simulink model "TorqueVect"  (R2022a)
settings: Solver=VariableStepAuto  StartTime=0.0  StopTime=32  RelTol=1e-3
PreLoadFcn:
  | run('Parameters\FSE_Parameters.m')
undefined symbols (not defined in the file): BRegenEnabledButton, canChannel, CyalphaLookUp, efficiency, Fz_curve, Fz_scaling_long, gearR, izz, jw, Kd, kd, Ki, ki, Kp, kp, l_f, l_r, lambda, m, Mz_max, N, N_lat, N_long, P_max, pid_kd_lat, pid_kd_long, pid_ki_lat, pid_ki_long, pid_kp_lat, pid_kp_long, R_max, rw, steerR, T_i_max, TC_Decr_Gas, TC_Derivative, TC_Incr_Gas, TC_On, TC_Relay_Off, TC_Relay_On, tireCornerStiffness, Ts, TV_On, TV_Override, velocity_lookup, velocity_lookup_lat, y_ref, yrr_scaling
libraries: simulink x218, slpidlib x135, CarMaker4SL x101, TractionControlLibrary x13, canmsglib x9, canlib x8, TorqueVectoringLibrary x6, simulink_extras x4, PedalConversionLibrary x3, PowerControlLibrary x1
(part 21 of 26)

== system TorqueVect/CarMaker/IPG Vehicle/PowerTrain/PTControl Example/PTControl_ALL_CTRL_VC_REGEN/Subsystem/TC/TractionControlFR/PID Controller ==
  rSlipError : Inport
  BEnable_TC : Inport  Port=2
  Kp_TC : Inport  Port=3
  Kd_TC : Inport  Port=4
  Ki_TC : Inport  Port=5
  MMotorMax : Inport  Port=6
  Constant : Constant  Value=0
  Constant1 : Constant  Value=0
  PID Controller : slpidlib/PID Controller  Controller=PID  Form=Ideal  TimeDomain=Discrete-time  UseExternalTs=off  SampleTime=0.005  IntegratorMethod=Forward Euler  FilterMethod=Forward Euler  ControllerParametersSource=external  P=Kp  I=Ki  UseKiTs=on  D=Kd  N=100  UseFilter=off  TunerSelectOption=Transfer Function Based (PID Tuner App)  InitialConditionSource=internal  InitialConditionForIntegrator=0  InitialConditionForFilter=0  DifferentiatorICPrevScaledInput=0  ExternalReset=either  TrackingMode=off  Kt=1  LimitOutput=on  SatLimitsSource=external  UpperSaturationLimit=21  LowerSaturationLimit=0  LinearizeAsGain=on  AntiWindupMode=none  Kb=1  POutMin=[]  POutMax=[]  IOutMin=[]  IOutMax=[]  DOutMin=[]  DOutMax=[]  NOutMin=[]  NOutMax=[]  SumOutMin=[]  SumOutMax=[]  SaturationOutMin=[]  SaturationOutMax=[]  PParamMin=[]  PParamMax=[]  IParamMin=[]  IParamMax=[]  DParamMin=[]  DParamMax=[]  NParamMin=[]  NParamMax=[]  KbParamMin=[]  KbParamMax=[]  KtParamMin=[]  KtParamMax=[]  KbOutMin=[]  KbOutMax=[]  KtOutMin=[]  KtOutMax=[]  IntegratorOutMin=[]  IntegratorOutMax=[]  FilterOutMin=[]  FilterOutMax=[]  SumI1OutMin=[]  SumI1OutMax=[]  SumI2OutMin=[]  SumI2OutMax=[]  SumI3OutMin=[]  SumI3OutMax=[]  SumI4OutMin=[]  SumI4OutMax=[]  SumDOutMin=[]  SumDOutMax=[]  DifferentiatorOutMin=[]  DifferentiatorOutMax=[]  FilterDiffOutCoefMin=[]  FilterDiffOutCoefMax=[]  ReciprocalOutMin=[]  ReciprocalOutMax=[]  SumDenOutMin=[]  SumDenOutMax=[]  SumNumOutMin=[]  SumNumOutMax=[]  DivideOutMin=[]  DivideOutMax=[]  UdiffTsProdOutMin=[]  UdiffTsProdOutMax=[]  NTsProdOutMin=[]  NTsProdOutMax=[]  UintegralTsProdOutMin=[]  UintegralTsProdOutMax=[]  UngainTsProdOutMin=[]  UngainTsProdOutMax=[]  ClampingZeroOutDataTypeStr=Inherit: Inherit via back propagation  ClampingZeroOutMin=[]  ClampingZeroOutMax=[]  FilterDenConstantOutDataTypeStr=Inherit: Inherit via back propagation  FilterDenConstantOutMin=[]  FilterDenConstantOutMax=[]  PCopyOutDataTypeStr=Inherit: Inherit via back propagation  PCopyOutMin=[]  PCopyOutMax=[]  NCopyOutDataTypeStr=Inherit: Inherit via back propagation  NCopyOutMin=[]  NCopyOutMax=[]  IntegratorContinuousStateAttributes=''  IntegratorStateMustResolveToSignalObject=off  IntegratorRTWStateStorageClass=Auto  FilterContinuousStateAttributes=''  FilterStateMustResolveToSignalObject=off  FilterRTWStateStorageClass=Auto  ParallelPVariant=Passthrough  IdealPVariant=ExternalParameters  IVariant=ExternalParameters  DVariant=ExternalParameters  IntegratorVariant=Discrete  SatVariant=External  AWVariant=Passthrough  PCopyVariant=Disabled  TRVariant=Disabled  FdbkBlocksVariant=Forward  IdealPFdbkVariant=Disabled  SatFdbkVariant=Disabled  DerivativeFilterVariant=Differentiator  NVariant=Passthrough  NCopyVariant=Disabled_SignalSpec  FilterICVariant=InternalICsDifferentiator  IntegratorICVariant=InternalICs  ExternalResetVariant=ExternalReset  TRSumVariant=Passthrough  SumFdbkVariant=Disabled  SumVariant=Sum_PID  TsampFilterVariant=InternalTs  TsampNgainVariant=Passthrough  TsampIntegralVariant=Passthrough  ExternalSaturationOutDataTypeStr=Inherit: Same as second input  aMode=0
  Switch : Switch  Criteria=u2 > Threshold  SaturateOnIntegerOverflow=off  InputSameDT=off
  MMotorReduction : Outport  VectorParamsAs1DForOutWhenUnconnected=off
  wires:
  Constant/1 -> Switch/3
  BEnable_TC/1 -> PID Controller/5, Switch/2
  Kp_TC/1 -> PID Controller/2
  rSlipError/1 -> PID Controller/1
  Kd_TC/1 -> PID Controller/4
  Switch/1 -> MMotorReduction/1
  Ki_TC/1 -> PID Controller/3
  Constant1/1 -> PID Controller/7
  MMotorMax/1 -> PID Controller/6
  PID Controller/1 -> Switch/1

== system TorqueVect/CarMaker/IPG Vehicle/PowerTrain/PTControl Example/PTControl_ALL_CTRL_VC_REGEN/Subsystem/TC/TractionControlRL/If Action Subsystem ==
  MMotorRequest : Inport
  Action Port : ActionPort
  Out1 : Outport
  wires:
  MMotorRequest/1 -> Out1/1

== system TorqueVect/CarMaker/IPG Vehicle/PowerTrain/PTControl Example/PTControl_ALL_CTRL_VC_REGEN/Subsystem/TC/TractionControlRL/If Action Subsystem1 ==
  Action Port : ActionPort
  Constant : Constant  Value=0
  Out1 : Outport
  wires:
  Constant/1 -> Out1/1

== system TorqueVect/CarMaker/IPG Vehicle/PowerTrain/PTControl Example/PTControl_ALL_CTRL_VC_REGEN/Subsystem/TC/TractionControlRL/If Action Subsystem2 ==
  MMotorRequest : Inport
  In2 : Inport  Port=2
  Action Port : ActionPort
  Add : Sum  Inputs=+-
  Out1 : Outport
  wires:
  In2/1 -> Add/2
  MMotorRequest/1 -> Add/1
  Add/1 -> Out1/1

== system TorqueVect/CarMaker/IPG Vehicle/PowerTrain/PTControl Example/PTControl_ALL_CTRL_VC_REGEN/Subsystem/TC/TractionControlRL/PID Controller ==
  rSlipError : Inport
  BEnable_TC : Inport  Port=2
  Kp_TC : Inport  Port=3
  Kd_TC : Inport  Port=4
  Ki_TC : Inport  Port=5
  MMotorMax : Inport  Port=6
  Constant : Constant  Value=0
  Constant1 : Constant  Value=0
  PID Controller : slpidlib/PID Controller  Controller=PID  Form=Ideal  TimeDomain=Discrete-time  UseExternalTs=off  SampleTime=0.005  IntegratorMethod=Forward Euler  FilterMethod=Forward Euler  ControllerParametersSource=external  P=Kp  I=Ki  UseKiTs=on  D=Kd  N=100  UseFilter=off  TunerSelectOption=Transfer Function Based (PID Tuner App)  InitialConditionSource=internal  InitialConditionForIntegrator=0  InitialConditionForFilter=0  DifferentiatorICPrevScaledInput=0  ExternalReset=either  TrackingMode=off  Kt=1  LimitOutput=on  SatLimitsSource=external  UpperSaturationLimit=21  LowerSaturationLimit=0  LinearizeAsGain=on  AntiWindupMode=none  Kb=1  POutMin=[]  POutMax=[]  IOutMin=[]  IOutMax=[]  DOutMin=[]  DOutMax=[]  NOutMin=[]  NOutMax=[]  SumOutMin=[]  SumOutMax=[]  SaturationOutMin=[]  SaturationOutMax=[]  PParamMin=[]  PParamMax=[]  IParamMin=[]  IParamMax=[]  DParamMin=[]  DParamMax=[]  NParamMin=[]  NParamMax=[]  KbParamMin=[]  KbParamMax=[]  KtParamMin=[]  KtParamMax=[]  KbOutMin=[]  KbOutMax=[]  KtOutMin=[]  KtOutMax=[]  IntegratorOutMin=[]  IntegratorOutMax=[]  FilterOutMin=[]  FilterOutMax=[]  SumI1OutMin=[]  SumI1OutMax=[]  SumI2OutMin=[]  SumI2OutMax=[]  SumI3OutMin=[]  SumI3OutMax=[]  SumI4OutMin=[]  SumI4OutMax=[]  SumDOutMin=[]  SumDOutMax=[]  DifferentiatorOutMin=[]  DifferentiatorOutMax=[]  FilterDiffOutCoefMin=[]  FilterDiffOutCoefMax=[]  ReciprocalOutMin=[]  ReciprocalOutMax=[]  SumDenOutMin=[]  SumDenOutMax=[]  SumNumOutMin=[]  SumNumOutMax=[]  DivideOutMin=[]  DivideOutMax=[]  UdiffTsProdOutMin=[]  UdiffTsProdOutMax=[]  NTsProdOutMin=[]  NTsProdOutMax=[]  UintegralTsProdOutMin=[]  UintegralTsProdOutMax=[]  UngainTsProdOutMin=[]  UngainTsProdOutMax=[]  ClampingZeroOutDataTypeStr=Inherit: Inherit via back propagation  ClampingZeroOutMin=[]  ClampingZeroOutMax=[]  FilterDenConstantOutDataTypeStr=Inherit: Inherit via back propagation  FilterDenConstantOutMin=[]  FilterDenConstantOutMax=[]  PCopyOutDataTypeStr=Inherit: Inherit via back propagation  PCopyOutMin=[]  PCopyOutMax=[]  NCopyOutDataTypeStr=Inherit: Inherit via back propagation  NCopyOutMin=[]  NCopyOutMax=[]  IntegratorContinuousStateAttributes=''  IntegratorStateMustResolveToSignalObject=off  IntegratorRTWStateStorageClass=Auto  FilterContinuousStateAttributes=''  FilterStateMustResolveToSignalObject=off  FilterRTWStateStorageClass=Auto  ParallelPVariant=Passthrough  IdealPVariant=ExternalParameters  IVariant=ExternalParameters  DVariant=ExternalParameters  IntegratorVariant=Discrete  SatVariant=External  AWVariant=Passthrough  PCopyVariant=Disabled  TRVariant=Disabled  FdbkBlocksVariant=Forward  IdealPFdbkVariant=Disabled  SatFdbkVariant=Disabled  DerivativeFilterVariant=Differentiator  NVariant=Passthrough  NCopyVariant=Disabled_SignalSpec  FilterICVariant=InternalICsDifferentiator  IntegratorICVariant=InternalICs  ExternalResetVariant=ExternalReset  TRSumVariant=Passthrough  SumFdbkVariant=Disabled  SumVariant=Sum_PID  TsampFilterVariant=InternalTs  TsampNgainVariant=Passthrough  TsampIntegralVariant=Passthrough  ExternalSaturationOutDataTypeStr=Inherit: Same as second input  aMode=0
  Switch : Switch  Criteria=u2 > Threshold  SaturateOnIntegerOverflow=off  InputSameDT=off
  MMotorReduction : Outport  VectorParamsAs1DForOutWhenUnconnected=off
  wires:
  Constant/1 -> Switch/3
  BEnable_TC/1 -> PID Controller/5, Switch/2
  Kp_TC/1 -> PID Controller/2
  rSlipError/1 -> PID Controller/1
  Kd_TC/1 -> PID Controller/4
  Switch/1 -> MMotorReduction/1
  Ki_TC/1 -> PID Controller/3
  Constant1/1 -> PID Controller/7
  MMotorMax/1 -> PID Controller/6
  PID Controller/1 -> Switch/1

== system TorqueVect/CarMaker/IPG Vehicle/PowerTrain/PTControl Example/PTControl_ALL_CTRL_VC_REGEN/Subsystem/TC/TractionControlRR/If Action Subsystem ==
  MMotorRequest : Inport
  Action Port : ActionPort
  Out1 : Outport
  wires:
  MMotorRequest/1 -> Out1/1

== system TorqueVect/CarMaker/IPG Vehicle/PowerTrain/PTControl Example/PTControl_ALL_CTRL_VC_REGEN/Subsystem/TC/TractionControlRR/If Action Subsystem1 ==
  Action Port : ActionPort
  Constant : Constant  Value=0
  Out1 : Outport
  wires:
  Constant/1 -> Out1/1

== system TorqueVect/CarMaker/IPG Vehicle/PowerTrain/PTControl Example/PTControl_ALL_CTRL_VC_REGEN/Subsystem/TC/TractionControlRR/If Action Subsystem2 ==
  MMotorRequest : Inport
  In2 : Inport  Port=2
  Action Port : ActionPort
  Add : Sum  Inputs=+-
  Out1 : Outport
  wires:
  In2/1 -> Add/2
  MMotorRequest/1 -> Add/1
  Add/1 -> Out1/1

== system TorqueVect/CarMaker/IPG Vehicle/PowerTrain/PTControl Example/PTControl_ALL_CTRL_VC_REGEN/Subsystem/TC/TractionControlRR/PID Controller ==
  rSlipError : Inport
  BEnable_TC : Inport  Port=2
  Kp_TC : Inport  Port=3
  Kd_TC : Inport  Port=4
  Ki_TC : Inport  Port=5
  MMotorMax : Inport  Port=6
  Constant : Constant  Value=0
  Constant1 : Constant  Value=0
  PID Controller : slpidlib/PID Controller  Controller=PID  Form=Ideal  TimeDomain=Discrete-time  UseExternalTs=off  SampleTime=0.005  IntegratorMethod=Forward Euler  FilterMethod=Forward Euler  ControllerParametersSource=external  P=Kp  I=Ki  UseKiTs=on  D=Kd  N=100  UseFilter=off  TunerSelectOption=Transfer Function Based (PID Tuner App)  InitialConditionSource=internal  InitialConditionForIntegrator=0  InitialConditionForFilter=0  DifferentiatorICPrevScaledInput=0  ExternalReset=either  TrackingMode=off  Kt=1  LimitOutput=on  SatLimitsSource=external  UpperSaturationLimit=21  LowerSaturationLimit=0  LinearizeAsGain=on  AntiWindupMode=none  Kb=1  POutMin=[]  POutMax=[]  IOutMin=[]  IOutMax=[]  DOutMin=[]  DOutMax=[]  NOutMin=[]  NOutMax=[]  SumOutMin=[]  SumOutMax=[]  SaturationOutMin=[]  SaturationOutMax=[]  PParamMin=[]  PParamMax=[]  IParamMin=[]  IParamMax=[]  DParamMin=[]  DParamMax=[]  NParamMin=[]  NParamMax=[]  KbParamMin=[]  KbParamMax=[]  KtParamMin=[]  KtParamMax=[]  KbOutMin=[]  KbOutMax=[]  KtOutMin=[]  KtOutMax=[]  IntegratorOutMin=[]  IntegratorOutMax=[]  FilterOutMin=[]  FilterOutMax=[]  SumI1OutMin=[]  SumI1OutMax=[]  SumI2OutMin=[]  SumI2OutMax=[]  SumI3OutMin=[]  SumI3OutMax=[]  SumI4OutMin=[]  SumI4OutMax=[]  SumDOutMin=[]  SumDOutMax=[]  DifferentiatorOutMin=[]  DifferentiatorOutMax=[]  FilterDiffOutCoefMin=[]  FilterDiffOutCoefMax=[]  ReciprocalOutMin=[]  ReciprocalOutMax=[]  SumDenOutMin=[]  SumDenOutMax=[]  SumNumOutMin=[]  SumNumOutMax=[]  DivideOutMin=[]  DivideOutMax=[]  UdiffTsProdOutMin=[]  UdiffTsProdOutMax=[]  NTsProdOutMin=[]  NTsProdOutMax=[]  UintegralTsProdOutMin=[]  UintegralTsProdOutMax=[]  UngainTsProdOutMin=[]  UngainTsProdOutMax=[]  ClampingZeroOutDataTypeStr=Inherit: Inherit via back propagation  ClampingZeroOutMin=[]  ClampingZeroOutMax=[]  FilterDenConstantOutDataTypeStr=Inherit: Inherit via back propagation  FilterDenConstantOutMin=[]  FilterDenConstantOutMax=[]  PCopyOutDataTypeStr=Inherit: Inherit via back propagation  PCopyOutMin=[]  PCopyOutMax=[]  NCopyOutDataTypeStr=Inherit: Inherit via back propagation  NCopyOutMin=[]  NCopyOutMax=[]  IntegratorContinuousStateAttributes=''  IntegratorStateMustResolveToSignalObject=off  IntegratorRTWStateStorageClass=Auto  FilterContinuousStateAttributes=''  FilterStateMustResolveToSignalObject=off  FilterRTWStateStorageClass=Auto  ParallelPVariant=Passthrough  IdealPVariant=ExternalParameters  IVariant=ExternalParameters  DVariant=ExternalParameters  IntegratorVariant=Discrete  SatVariant=External  AWVariant=Passthrough  PCopyVariant=Disabled  TRVariant=Disabled  FdbkBlocksVariant=Forward  IdealPFdbkVariant=Disabled  SatFdbkVariant=Disabled  DerivativeFilterVariant=Differentiator  NVariant=Passthrough  NCopyVariant=Disabled_SignalSpec  FilterICVariant=InternalICsDifferentiator  IntegratorICVariant=InternalICs  ExternalResetVariant=ExternalReset  TRSumVariant=Passthrough  SumFdbkVariant=Disabled  SumVariant=Sum_PID  TsampFilterVariant=InternalTs  TsampNgainVariant=Passthrough  TsampIntegralVariant=Passthrough  ExternalSaturationOutDataTypeStr=Inherit: Same as second input  aMode=0
  Switch : Switch  Criteria=u2 > Threshold  SaturateOnIntegerOverflow=off  InputSameDT=off
  MMotorReduction : Outport  VectorParamsAs1DForOutWhenUnconnected=off
  wires:
  Constant/1 -> Switch/3
  BEnable_TC/1 -> PID Controller/5, Switch/2
  Kp_TC/1 -> PID Controller/2
  rSlipError/1 -> PID Controller/1
  Kd_TC/1 -> PID Controller/4
  Switch/1 -> MMotorReduction/1
  Ki_TC/1 -> PID Controller/3
  Constant1/1 -> PID Controller/7
  MMotorMax/1 -> PID Controller/6
  PID Controller/1 -> Switch/1

== system TorqueVect/CarMaker/IPG Vehicle/PowerTrain/PTControl Example/PTControl_ALL_CTRL_VC_REGEN/Subsystem/Torque Vectoring/FPID/If Action Subsystem ==
  NTorqueWheel : Inport
  NTorqueDelta : Inport  Port=2
  Add : Sum  Inputs=+-
  Add1 : Sum
  NTorqueLeftOut : Outport
  NTorqueRightOut : Outport  Port=2
  wires:
  Add/1 -> NTorqueLeftOut/1
  Add1/1 -> NTorqueRightOut/1
  NTorqueWheel/1 -> Add1/1, Add/1
  NTorqueDelta/1 -> Add1/2, Add/2

== system TorqueVect/CarMaker/IPG Vehicle/PowerTrain/PTControl Example/PTControl_ALL_CTRL_VC_REGEN/Subsystem/Torque Vectoring/RPID/If Action Subsystem ==
  NTorqueWheel : Inport
  NTorqueDelta : Inport  Port=2
  Add : Sum  Inputs=+-
  Add1 : Sum
  NTorqueLeftOut : Outport
  NTorqueRightOut : Outport  Port=2
  wires:
  Add/1 -> NTorqueLeftOut/1
  Add1/1 -> NTorqueRightOut/1
  NTorqueWheel/1 -> Add1/1, Add/1
  NTorqueDelta/1 -> Add1/2, Add/2

== system TorqueVect/CarMaker/IPG Vehicle/PowerTrain/PTControl Example/PTControl_ALL_CTRL_VC_REGEN/Subsystem1/TC/TractionControlFL/If Action Subsystem ==
  MMotorRequest : Inport
  Action Port : ActionPort
  Out1 : Outport
  wires:
  MMotorRequest/1 -> Out1/1

== system TorqueVect/CarMaker/IPG Vehicle/PowerTrain/PTControl Example/PTControl_ALL_CTRL_VC_REGEN/Subsystem1/TC/TractionControlFL/If Action Subsystem1 ==
  Action Port : ActionPort
  Constant : Constant  Value=0
  Out1 : Outport
  wires:
  Constant/1 -> Out1/1

== system TorqueVect/CarMaker/IPG Vehicle/PowerTrain/PTControl Example/PTControl_ALL_CTRL_VC_REGEN/Subsystem1/TC/TractionControlFL/If Action Subsystem2 ==
  MMotorRequest : Inport
  In2 : Inport  Port=2
  Action Port : ActionPort
  Add : Sum  Inputs=+-
  Out1 : Outport
  wires:
  In2/1 -> Add/2
  MMotorRequest/1 -> Add/1
  Add/1 -> Out1/1

== system TorqueVect/CarMaker/IPG Vehicle/PowerTrain/PTControl Example/PTControl_ALL_CTRL_VC_REGEN/Subsystem1/TC/TractionControlFL/PID Controller ==
  rSlipError : Inport
  BEnable_TC : Inport  Port=2
  Kp_TC : Inport  Port=3
  Kd_TC : Inport  Port=4
  Ki_TC : Inport  Port=5
  MMotorMax : Inport  Port=6
  resetTC : Inport  Port=7
  Constant : Constant  Value=0
  Constant1 : Constant  Value=0
  OR : Logic  Operator=OR  IconShape=distinctive  AllPortsSameDT=off  OutDataTypeStr=boolean
  PID Controller : slpidlib/PID Controller  Controller=PID  Form=Ideal  TimeDomain=Discrete-time  UseExternalTs=off  SampleTime=0.005  IntegratorMethod=Forward Euler  FilterMethod=Forward Euler  ControllerParametersSource=external  P=Kp  I=Ki  UseKiTs=on  D=Kd  N=100  UseFilter=off  TunerSelectOption=Transfer Function Based (PID Tuner App)  InitialConditionSource=internal  InitialConditionForIntegrator=0  InitialConditionForFilter=0  DifferentiatorICPrevScaledInput=0  ExternalReset=either  TrackingMode=off  Kt=1  LimitOutput=on  SatLimitsSource=external  UpperSaturationLimit=21  LowerSaturationLimit=0  LinearizeAsGain=on  AntiWindupMode=none  Kb=1  POutMin=[]  POutMax=[]  IOutMin=[]  IOutMax=[]  DOutMin=[]  DOutMax=[]  NOutMin=[]  NOutMax=[]  SumOutMin=[]  SumOutMax=[]  SaturationOutMin=[]  SaturationOutMax=[]  PParamMin=[]  PParamMax=[]  IParamMin=[]  IParamMax=[]  DParamMin=[]  DParamMax=[]  NParamMin=[]  NParamMax=[]  KbParamMin=[]  KbParamMax=[]  KtParamMin=[]  KtParamMax=[]  KbOutMin=[]  KbOutMax=[]  KtOutMin=[]  KtOutMax=[]  IntegratorOutMin=[]  IntegratorOutMax=[]  FilterOutMin=[]  FilterOutMax=[]  SumI1OutMin=[]  SumI1OutMax=[]  SumI2OutMin=[]  SumI2OutMax=[]  SumI3OutMin=[]  SumI3OutMax=[]  SumI4OutMin=[]  SumI4OutMax=[]  SumDOutMin=[]  SumDOutMax=[]  DifferentiatorOutMin=[]  DifferentiatorOutMax=[]  FilterDiffOutCoefMin=[]  FilterDiffOutCoefMax=[]  ReciprocalOutMin=[]  ReciprocalOutMax=[]  SumDenOutMin=[]  SumDenOutMax=[]  SumNumOutMin=[]  SumNumOutMax=[]  DivideOutMin=[]  DivideOutMax=[]  UdiffTsProdOutMin=[]  UdiffTsProdOutMax=[]  NTsProdOutMin=[]  NTsProdOutMax=[]  UintegralTsProdOutMin=[]  UintegralTsProdOutMax=[]  UngainTsProdOutMin=[]  UngainTsProdOutMax=[]  ClampingZeroOutDataTypeStr=Inherit: Inherit via back propagation  ClampingZeroOutMin=[]  ClampingZeroOutMax=[]  FilterDenConstantOutDataTypeStr=Inherit: Inherit via back propagation  FilterDenConstantOutMin=[]  FilterDenConstantOutMax=[]  PCopyOutDataTypeStr=Inherit: Inherit via back propagation  PCopyOutMin=[]  PCopyOutMax=[]  NCopyOutDataTypeStr=Inherit: Inherit via back propagation  NCopyOutMin=[]  NCopyOutMax=[]  IntegratorContinuousStateAttributes=''  IntegratorStateMustResolveToSignalObject=off  IntegratorRTWStateStorageClass=Auto  FilterContinuousStateAttributes=''  FilterStateMustResolveToSignalObject=off  FilterRTWStateStorageClass=Auto  ParallelPVariant=Passthrough  IdealPVariant=ExternalParameters  IVariant=ExternalParameters  DVariant=ExternalParameters  IntegratorVariant=Discrete  SatVariant=External  AWVariant=Passthrough  PCopyVariant=Disabled  TRVariant=Disabled  FdbkBlocksVariant=Forward  IdealPFdbkVariant=Disabled  SatFdbkVariant=Disabled  DerivativeFilterVariant=Differentiator  NVariant=Passthrough  NCopyVariant=Disabled_SignalSpec  FilterICVariant=InternalICsDifferentiator  IntegratorICVariant=InternalICs  ExternalResetVariant=ExternalReset  TRSumVariant=Passthrough  SumFdbkVariant=Disabled  SumVariant=Sum_PID  TsampFilterVariant=InternalTs  TsampNgainVariant=Passthrough  TsampIntegralVariant=Passthrough  ExternalSaturationOutDataTypeStr=Inherit: Same as second input  aMode=0
  Switch : Switch  Criteria=u2 > Threshold  SaturateOnIntegerOverflow=off  InputSameDT=off
  MMotorReduction : Outport  VectorParamsAs1DForOutWhenUnconnected=off
  wires:
  Constant/1 -> Switch/3
  PID Controller/1 -> Switch/1
  Kp_TC/1 -> PID Controller/2
  rSlipError/1 -> PID Controller/1
  Kd_TC/1 -> PID Controller/4
  Switch/1 -> MMotorReduction/1
  Ki_TC/1 -> PID Controller/3
  Constant1/1 -> PID Controller/7
  MMotorMax/1 -> PID Controller/6
  OR/1 -> PID Controller/5
  resetTC/1 -> OR/2
  BEnable_TC/1 -> Switch/2, OR/1

== system TorqueVect/CarMaker/IPG Vehicle/PowerTrain/PTControl Example/PTControl_ALL_CTRL_VC_REGEN/Subsystem1/TC/TractionControlFR/If Action Subsystem ==
  MMotorRequest : Inport
  Action Port : ActionPort
  Out1 : Outport
  wires:
  MMotorRequest/1 -> Out1/1

== system TorqueVect/CarMaker/IPG Vehicle/PowerTrain/PTControl Example/PTControl_ALL_CTRL_VC_REGEN/Subsystem1/TC/TractionControlFR/If Action Subsystem1 ==
  Action Port : ActionPort
  Constant : Constant  Value=0
  Out1 : Outport
  wires:
  Constant/1 -> Out1/1

== system TorqueVect/CarMaker/IPG Vehicle/PowerTrain/PTControl Example/PTControl_ALL_CTRL_VC_REGEN/Subsystem1/TC/TractionControlFR/If Action Subsystem2 ==
  MMotorRequest : Inport
  In2 : Inport  Port=2
  Action Port : ActionPort
  Add : Sum  Inputs=+-
  Out1 : Outport
  wires:
  In2/1 -> Add/2
  MMotorRequest/1 -> Add/1
  Add/1 -> Out1/1

== system TorqueVect/CarMaker/IPG Vehicle/PowerTrain/PTControl Example/PTControl_ALL_CTRL_VC_REGEN/Subsystem1/TC/TractionControlFR/PID Controller ==
  rSlipError : Inport
  BEnable_TC : Inport  Port=2
  Kp_TC : Inport  Port=3
  Kd_TC : Inport  Port=4
  Ki_TC : Inport  Port=5
  MMotorMax : Inport  Port=6
  resetTC : Inport  Port=7
  Constant : Constant  Value=0
  Constant1 : Constant  Value=0
  OR : Logic  Operator=OR  IconShape=distinctive  AllPortsSameDT=off  OutDataTypeStr=boolean
  PID Controller : slpidlib/PID Controller  Controller=PID  Form=Ideal  TimeDomain=Discrete-time  UseExternalTs=off  SampleTime=0.005  IntegratorMethod=Forward Euler  FilterMethod=Forward Euler  ControllerParametersSource=external  P=Kp  I=Ki  UseKiTs=on  D=Kd  N=100  UseFilter=off  TunerSelectOption=Transfer Function Based (PID Tuner App)  InitialConditionSource=internal  InitialConditionForIntegrator=0  InitialConditionForFilter=0  DifferentiatorICPrevScaledInput=0  ExternalReset=either  TrackingMode=off  Kt=1  LimitOutput=on  SatLimitsSource=external  UpperSaturationLimit=21  LowerSaturationLimit=0  LinearizeAsGain=on  AntiWindupMode=none  Kb=1  POutMin=[]  POutMax=[]  IOutMin=[]  IOutMax=[]  DOutMin=[]  DOutMax=[]  NOutMin=[]  NOutMax=[]  SumOutMin=[]  SumOutMax=[]  SaturationOutMin=[]  SaturationOutMax=[]  PParamMin=[]  PParamMax=[]  IParamMin=[]  IParamMax=[]  DParamMin=[]  DParamMax=[]  NParamMin=[]  NParamMax=[]  KbParamMin=[]  KbParamMax=[]  KtParamMin=[]  KtParamMax=[]  KbOutMin=[]  KbOutMax=[]  KtOutMin=[]  KtOutMax=[]  IntegratorOutMin=[]  IntegratorOutMax=[]  FilterOutMin=[]  FilterOutMax=[]  SumI1OutMin=[]  SumI1OutMax=[]  SumI2OutMin=[]  SumI2OutMax=[]  SumI3OutMin=[]  SumI3OutMax=[]  SumI4OutMin=[]  SumI4OutMax=[]  SumDOutMin=[]  SumDOutMax=[]  DifferentiatorOutMin=[]  DifferentiatorOutMax=[]  FilterDiffOutCoefMin=[]  FilterDiffOutCoefMax=[]  ReciprocalOutMin=[]  ReciprocalOutMax=[]  SumDenOutMin=[]  SumDenOutMax=[]  SumNumOutMin=[]  SumNumOutMax=[]  DivideOutMin=[]  DivideOutMax=[]  UdiffTsProdOutMin=[]  UdiffTsProdOutMax=[]  NTsProdOutMin=[]  NTsProdOutMax=[]  UintegralTsProdOutMin=[]  UintegralTsProdOutMax=[]  UngainTsProdOutMin=[]  UngainTsProdOutMax=[]  ClampingZeroOutDataTypeStr=Inherit: Inherit via back propagation  ClampingZeroOutMin=[]  ClampingZeroOutMax=[]  FilterDenConstantOutDataTypeStr=Inherit: Inherit via back propagation  FilterDenConstantOutMin=[]  FilterDenConstantOutMax=[]  PCopyOutDataTypeStr=Inherit: Inherit via back propagation  PCopyOutMin=[]  PCopyOutMax=[]  NCopyOutDataTypeStr=Inherit: Inherit via back propagation  NCopyOutMin=[]  NCopyOutMax=[]  IntegratorContinuousStateAttributes=''  IntegratorStateMustResolveToSignalObject=off  IntegratorRTWStateStorageClass=Auto  FilterContinuousStateAttributes=''  FilterStateMustResolveToSignalObject=off  FilterRTWStateStorageClass=Auto  ParallelPVariant=Passthrough  IdealPVariant=ExternalParameters  IVariant=ExternalParameters  DVariant=ExternalParameters  IntegratorVariant=Discrete  SatVariant=External  AWVariant=Passthrough  PCopyVariant=Disabled  TRVariant=Disabled  FdbkBlocksVariant=Forward  IdealPFdbkVariant=Disabled  SatFdbkVariant=Disabled  DerivativeFilterVariant=Differentiator  NVariant=Passthrough  NCopyVariant=Disabled_SignalSpec  FilterICVariant=InternalICsDifferentiator  IntegratorICVariant=InternalICs  ExternalResetVariant=ExternalReset  TRSumVariant=Passthrough  SumFdbkVariant=Disabled  SumVariant=Sum_PID  TsampFilterVariant=InternalTs  TsampNgainVariant=Passthrough  TsampIntegralVariant=Passthrough  ExternalSaturationOutDataTypeStr=Inherit: Same as second input  aMode=0
  Switch : Switch  Criteria=u2 > Threshold  SaturateOnIntegerOverflow=off  InputSameDT=off
  MMotorReduction : Outport  VectorParamsAs1DForOutWhenUnconnected=off
  wires:
  Constant/1 -> Switch/3
  Kp_TC/1 -> PID Controller/2
  rSlipError/1 -> PID Controller/1
  Kd_TC/1 -> PID Controller/4
  Switch/1 -> MMotorReduction/1
  Ki_TC/1 -> PID Controller/3
  Constant1/1 -> PID Controller/7
  MMotorMax/1 -> PID Controller/6
  PID Controller/1 -> Switch/1
  resetTC/1 -> OR/2
  OR/1 -> PID Controller/5
  BEnable_TC/1 -> Switch/2, OR/1

== system TorqueVect/CarMaker/IPG Vehicle/PowerTrain/PTControl Example/PTControl_ALL_CTRL_VC_REGEN/Subsystem1/TC/TractionControlRL/If Action Subsystem ==
  MMotorRequest : Inport
  Action Port : ActionPort
  Out1 : Outport
  wires:
  MMotorRequest/1 -> Out1/1

== system TorqueVect/CarMaker/IPG Vehicle/PowerTrain/PTControl Example/PTControl_ALL_CTRL_VC_REGEN/Subsystem1/TC/TractionControlRL/If Action Subsystem1 ==
  Action Port : ActionPort
  Constant : Constant  Value=0
  Out1 : Outport
  wires:
  Constant/1 -> Out1/1

== system TorqueVect/CarMaker/IPG Vehicle/PowerTrain/PTControl Example/PTControl_ALL_CTRL_VC_REGEN/Subsystem1/TC/TractionControlRL/If Action Subsystem2 ==
  MMotorRequest : Inport
  In2 : Inport  Port=2
  Action Port : ActionPort
  Add : Sum  Inputs=+-
  Out1 : Outport
  wires:
  In2/1 -> Add/2
  MMotorRequest/1 -> Add/1
  Add/1 -> Out1/1

== system TorqueVect/CarMaker/IPG Vehicle/PowerTrain/PTControl Example/PTControl_ALL_CTRL_VC_REGEN/Subsystem1/TC/TractionControlRL/PID Controller ==
  rSlipError : Inport
  BEnable_TC : Inport  Port=2
  Kp_TC : Inport  Port=3
  Kd_TC : Inport  Port=4
  Ki_TC : Inport  Port=5
  MMotorMax : Inport  Port=6
  resetTC : Inport  Port=7
  Constant : Constant  Value=0
  Constant1 : Constant  Value=0
  OR : Logic  Operator=OR  IconShape=distinctive  AllPortsSameDT=off  OutDataTypeStr=boolean
  PID Controller : slpidlib/PID Controller  Controller=PID  Form=Ideal  TimeDomain=Discrete-time  UseExternalTs=off  SampleTime=0.005  IntegratorMethod=Forward Euler  FilterMethod=Forward Euler  ControllerParametersSource=external  P=Kp  I=Ki  UseKiTs=on  D=Kd  N=100  UseFilter=off  TunerSelectOption=Transfer Function Based (PID Tuner App)  InitialConditionSource=internal  InitialConditionForIntegrator=0  InitialConditionForFilter=0  DifferentiatorICPrevScaledInput=0  ExternalReset=either  TrackingMode=off  Kt=1  LimitOutput=on  SatLimitsSource=external  UpperSaturationLimit=21  LowerSaturationLimit=0  LinearizeAsGain=on  AntiWindupMode=none  Kb=1  POutMin=[]  POutMax=[]  IOutMin=[]  IOutMax=[]  DOutMin=[]  DOutMax=[]  NOutMin=[]  NOutMax=[]  SumOutMin=[]  SumOutMax=[]  SaturationOutMin=[]  SaturationOutMax=[]  PParamMin=[]  PParamMax=[]  IParamMin=[]  IParamMax=[]  DParamMin=[]  DParamMax=[]  NParamMin=[]  NParamMax=[]  KbParamMin=[]  KbParamMax=[]  KtParamMin=[]  KtParamMax=[]  KbOutMin=[]  KbOutMax=[]  KtOutMin=[]  KtOutMax=[]  IntegratorOutMin=[]  IntegratorOutMax=[]  FilterOutMin=[]  FilterOutMax=[]  SumI1OutMin=[]  SumI1OutMax=[]  SumI2OutMin=[]  SumI2OutMax=[]  SumI3OutMin=[]  SumI3OutMax=[]  SumI4OutMin=[]  SumI4OutMax=[]  SumDOutMin=[]  SumDOutMax=[]  DifferentiatorOutMin=[]  DifferentiatorOutMax=[]  FilterDiffOutCoefMin=[]  FilterDiffOutCoefMax=[]  ReciprocalOutMin=[]  ReciprocalOutMax=[]  SumDenOutMin=[]  SumDenOutMax=[]  SumNumOutMin=[]  SumNumOutMax=[]  DivideOutMin=[]  DivideOutMax=[]  UdiffTsProdOutMin=[]  UdiffTsProdOutMax=[]  NTsProdOutMin=[]  NTsProdOutMax=[]  UintegralTsProdOutMin=[]  UintegralTsProdOutMax=[]  UngainTsProdOutMin=[]  UngainTsProdOutMax=[]  ClampingZeroOutDataTypeStr=Inherit: Inherit via back propagation  ClampingZeroOutMin=[]  ClampingZeroOutMax=[]  FilterDenConstantOutDataTypeStr=Inherit: Inherit via back propagation  FilterDenConstantOutMin=[]  FilterDenConstantOutMax=[]  PCopyOutDataTypeStr=Inherit: Inherit via back propagation  PCopyOutMin=[]  PCopyOutMax=[]  NCopyOutDataTypeStr=Inherit: Inherit via back propagation  NCopyOutMin=[]  NCopyOutMax=[]  IntegratorContinuousStateAttributes=''  IntegratorStateMustResolveToSignalObject=off  IntegratorRTWStateStorageClass=Auto  FilterContinuousStateAttributes=''  FilterStateMustResolveToSignalObject=off  FilterRTWStateStorageClass=Auto  ParallelPVariant=Passthrough  IdealPVariant=ExternalParameters  IVariant=ExternalParameters  DVariant=ExternalParameters  IntegratorVariant=Discrete  SatVariant=External  AWVariant=Passthrough  PCopyVariant=Disabled  TRVariant=Disabled  FdbkBlocksVariant=Forward  IdealPFdbkVariant=Disabled  SatFdbkVariant=Disabled  DerivativeFilterVariant=Differentiator  NVariant=Passthrough  NCopyVariant=Disabled_SignalSpec  FilterICVariant=InternalICsDifferentiator  IntegratorICVariant=InternalICs  ExternalResetVariant=ExternalReset  TRSumVariant=Passthrough  SumFdbkVariant=Disabled  SumVariant=Sum_PID  TsampFilterVariant=InternalTs  TsampNgainVariant=Passthrough  TsampIntegralVariant=Passthrough  ExternalSaturationOutDataTypeStr=Inherit: Same as second input  aMode=0
  Switch : Switch  Criteria=u2 > Threshold  SaturateOnIntegerOverflow=off  InputSameDT=off
  MMotorReduction : Outport  VectorParamsAs1DForOutWhenUnconnected=off
  wires:
  Constant/1 -> Switch/3
  Kp_TC/1 -> PID Controller/2
  rSlipError/1 -> PID Controller/1
  Kd_TC/1 -> PID Controller/4
  Switch/1 -> MMotorReduction/1
  Ki_TC/1 -> PID Controller/3
  Constant1/1 -> PID Controller/7
  MMotorMax/1 -> PID Controller/6
  PID Controller/1 -> Switch/1
  resetTC/1 -> OR/2
  BEnable_TC/1 -> Switch/2, OR/1
  OR/1 -> PID Controller/5

== system TorqueVect/CarMaker/IPG Vehicle/PowerTrain/PTControl Example/PTControl_ALL_CTRL_VC_REGEN/Subsystem1/TC/TractionControlRR/If Action Subsystem ==
  MMotorRequest : Inport
  Action Port : ActionPort
  Out1 : Outport
  wires:
  MMotorRequest/1 -> Out1/1

== system TorqueVect/CarMaker/IPG Vehicle/PowerTrain/PTControl Example/PTControl_ALL_CTRL_VC_REGEN/Subsystem1/TC/TractionControlRR/If Action Subsystem1 ==
  Action Port : ActionPort
  Constant : Constant  Value=0
  Out1 : Outport
  wires:
  Constant/1 -> Out1/1

== system TorqueVect/CarMaker/IPG Vehicle/PowerTrain/PTControl Example/PTControl_ALL_CTRL_VC_REGEN/Subsystem1/TC/TractionControlRR/If Action Subsystem2 ==
  MMotorRequest : Inport
  In2 : Inport  Port=2
  Action Port : ActionPort
  Add : Sum  Inputs=+-
  Out1 : Outport
  wires:
  In2/1 -> Add/2
  MMotorRequest/1 -> Add/1
  Add/1 -> Out1/1

== system TorqueVect/CarMaker/IPG Vehicle/PowerTrain/PTControl Example/PTControl_ALL_CTRL_VC_REGEN/Subsystem1/TC/TractionControlRR/PID Controller ==
  rSlipError : Inport
  BEnable_TC : Inport  Port=2
  Kp_TC : Inport  Port=3
  Kd_TC : Inport  Port=4
  Ki_TC : Inport  Port=5
  MMotorMax : Inport  Port=6
  resetTC : Inport  Port=7
  Constant : Constant  Value=0
  Constant1 : Constant  Value=0
  OR : Logic  Operator=OR  IconShape=distinctive  AllPortsSameDT=off  OutDataTypeStr=boolean
  PID Controller : slpidlib/PID Controller  Controller=PID  Form=Ideal  TimeDomain=Discrete-time  UseExternalTs=off  SampleTime=0.005  IntegratorMethod=Forward Euler  FilterMethod=Forward Euler  ControllerParametersSource=external  P=Kp  I=Ki  UseKiTs=on  D=Kd  N=100  UseFilter=off  TunerSelectOption=Transfer Function Based (PID Tuner App)  InitialConditionSource=internal  InitialConditionForIntegrator=0  InitialConditionForFilter=0  DifferentiatorICPrevScaledInput=0  ExternalReset=either  TrackingMode=off  Kt=1  LimitOutput=on  SatLimitsSource=external  UpperSaturationLimit=21  LowerSaturationLimit=0  LinearizeAsGain=on  AntiWindupMode=none  Kb=1  POutMin=[]  POutMax=[]  IOutMin=[]  IOutMax=[]  DOutMin=[]  DOutMax=[]  NOutMin=[]  NOutMax=[]  SumOutMin=[]  SumOutMax=[]  SaturationOutMin=[]  SaturationOutMax=[]  PParamMin=[]  PParamMax=[]  IParamMin=[]  IParamMax=[]  DParamMin=[]  DParamMax=[]  NParamMin=[]  NParamMax=[]  KbParamMin=[]  KbParamMax=[]  KtParamMin=[]  KtParamMax=[]  KbOutMin=[]  KbOutMax=[]  KtOutMin=[]  KtOutMax=[]  IntegratorOutMin=[]  IntegratorOutMax=[]  FilterOutMin=[]  FilterOutMax=[]  SumI1OutMin=[]  SumI1OutMax=[]  SumI2OutMin=[]  SumI2OutMax=[]  SumI3OutMin=[]  SumI3OutMax=[]  SumI4OutMin=[]  SumI4OutMax=[]  SumDOutMin=[]  SumDOutMax=[]  DifferentiatorOutMin=[]  DifferentiatorOutMax=[]  FilterDiffOutCoefMin=[]  FilterDiffOutCoefMax=[]  ReciprocalOutMin=[]  ReciprocalOutMax=[]  SumDenOutMin=[]  SumDenOutMax=[]  SumNumOutMin=[]  SumNumOutMax=[]  DivideOutMin=[]  DivideOutMax=[]  UdiffTsProdOutMin=[]  UdiffTsProdOutMax=[]  NTsProdOutMin=[]  NTsProdOutMax=[]  UintegralTsProdOutMin=[]  UintegralTsProdOutMax=[]  UngainTsProdOutMin=[]  UngainTsProdOutMax=[]  ClampingZeroOutDataTypeStr=Inherit: Inherit via back propagation  ClampingZeroOutMin=[]  ClampingZeroOutMax=[]  FilterDenConstantOutDataTypeStr=Inherit: Inherit via back propagation  FilterDenConstantOutMin=[]  FilterDenConstantOutMax=[]  PCopyOutDataTypeStr=Inherit: Inherit via back propagation  PCopyOutMin=[]  PCopyOutMax=[]  NCopyOutDataTypeStr=Inherit: Inherit via back propagation  NCopyOutMin=[]  NCopyOutMax=[]  IntegratorContinuousStateAttributes=''  IntegratorStateMustResolveToSignalObject=off  IntegratorRTWStateStorageClass=Auto  FilterContinuousStateAttributes=''  FilterStateMustResolveToSignalObject=off  FilterRTWStateStorageClass=Auto  ParallelPVariant=Passthrough  IdealPVariant=ExternalParameters  IVariant=ExternalParameters  DVariant=ExternalParameters  IntegratorVariant=Discrete  SatVariant=External  AWVariant=Passthrough  PCopyVariant=Disabled  TRVariant=Disabled  FdbkBlocksVariant=Forward  IdealPFdbkVariant=Disabled  SatFdbkVariant=Disabled  DerivativeFilterVariant=Differentiator  NVariant=Passthrough  NCopyVariant=Disabled_SignalSpec  FilterICVariant=InternalICsDifferentiator  IntegratorICVariant=InternalICs  ExternalResetVariant=ExternalReset  TRSumVariant=Passthrough  SumFdbkVariant=Disabled  SumVariant=Sum_PID  TsampFilterVariant=InternalTs  TsampNgainVariant=Passthrough  TsampIntegralVariant=Passthrough  ExternalSaturationOutDataTypeStr=Inherit: Same as second input  aMode=0
  Switch : Switch  Criteria=u2 > Threshold  SaturateOnIntegerOverflow=off  InputSameDT=off
  MMotorReduction : Outport  VectorParamsAs1DForOutWhenUnconnected=off
  wires:
  Constant/1 -> Switch/3
  BEnable_TC/1 -> OR/1, Switch/2
  Kp_TC/1 -> PID Controller/2
  rSlipError/1 -> PID Controller/1
  Kd_TC/1 -> PID Controller/4
  Switch/1 -> MMotorReduction/1
  Ki_TC/1 -> PID Controller/3
  Constant1/1 -> PID Controller/7
  MMotorMax/1 -> PID Controller/6
  PID Controller/1 -> Switch/1
  OR/1 -> PID Controller/5
  resetTC/1 -> OR/2

== system TorqueVect/CarMaker/IPG Vehicle/PowerTrain/PTControl Example/PTControl_ALL_CTRL_VC_REGEN/Subsystem1/Torque Vectoring/F PID/If Action Subsystem ==
  NTorqueWheel : Inport
  NTorqueDelta : Inport  Port=2
  Action Port : ActionPort
  Add : Sum  Inputs=+-
  Add1 : Sum
  NTorqueLeftOut : Outport
  NTorqueRightOut : Outport  Port=2
  wires:
  Add/1 -> NTorqueLeftOut/1
  Add1/1 -> NTorqueRightOut/1
  NTorqueWheel/1 -> Add1/1, Add/1
  NTorqueDelta/1 -> Add1/2, Add/2

== system TorqueVect/CarMaker/IPG Vehicle/PowerTrain/PTControl Example/PTControl_ALL_CTRL_VC_REGEN/Subsystem1/Torque Vectoring/F PID/If Action Subsystem1 ==
  NTorqueWheel : Inport
  Action Port : ActionPort
  NTorqueLeftOut : Outport
  NTorqueRightOut : Outport  Port=2
  wires:
  NTorqueWheel/1 -> NTorqueRightOut/1, NTorqueLeftOut/1

== system TorqueVect/CarMaker/IPG Vehicle/PowerTrain/PTControl Example/PTControl_ALL_CTRL_VC_REGEN/Subsystem1/Torque Vectoring/R PID/If Action Subsystem ==
  NTorqueWheel : Inport
  NTorqueDelta : Inport  Port=2
  Action Port : ActionPort
  Add : Sum  Inputs=+-
  Add1 : Sum
  NTorqueLeftOut : Outport
  NTorqueRightOut : Outport  Port=2
  wires:
  Add/1 -> NTorqueLeftOut/1
  Add1/1 -> NTorqueRightOut/1
  NTorqueWheel/1 -> Add1/1, Add/1
  NTorqueDelta/1 -> Add1/2, Add/2

== system TorqueVect/CarMaker/IPG Vehicle/PowerTrain/PTControl Example/PTControl_ALL_CTRL_VC_REGEN/Subsystem1/Torque Vectoring/R PID/If Action Subsystem1 ==
  NTorqueWheel : Inport
  Action Port : ActionPort
  NTorqueLeftOut : Outport
  NTorqueRightOut : Outport  Port=2
  wires:
  NTorqueWheel/1 -> NTorqueRightOut/1, NTorqueLeftOut/1

== system TorqueVect/CarMaker/IPG Vehicle/PowerTrain/PTControl Example/PTControl_ALL_Speedgoat/New TC/TC R1/traction_controller/traction_controller ==
  dslip : Inport
  enable_tc : Inport  Port=2
  Kp : Inport  Port=3
  Kd : Inport  Port=4
  Constant : Constant  Value=0
  GreaterThan : RelationalOperator  Operator=>  OutDataTypeStr=boolean  RndMeth=Simplest  InputSameDT=off
  Merge : Merge
  PD Controller : Subsystem  TreatAsAtomicUnit=on
  default : Subsystem  TreatAsAtomicUnit=on
  if_below_target_sr : If  IfExpression=u1 == 0
  delta_torque : Outport  VectorParamsAs1DForOutWhenUnconnected=off
  wires:
  Merge/1 -> delta_torque/1
  default/1(no_change) -> Merge/1
  PD Controller/1(delta_torque) -> Merge/2
  dslip/1 -> PD Controller/1(dslip), GreaterThan/1
  enable_tc/1 -> PD Controller/2(enable_tc)
  Kp/1 -> PD Controller/3(Kp)
  Kd/1 -> PD Controller/4(Kd)
  GreaterThan/1 -> if_below_target_sr/1
  Constant/1 -> GreaterThan/2
  if_below_target_sr/1 -> default/Action
  if_below_target_sr/2 -> PD Controller/Action

== system TorqueVect/CarMaker/IPG Vehicle/PowerTrain/PTControl Example/PTControl_ALL_Speedgoat/New TC/TC R2/traction_controller/traction_controller ==
  dslip : Inport
  enable_tc : Inport  Port=2
  Kp : Inport  Port=3
  Kd : Inport  Port=4
  Constant : Constant  Value=0
  GreaterThan : RelationalOperator  Operator=>  OutDataTypeStr=boolean  RndMeth=Simplest  InputSameDT=off
  Merge : Merge
  PD Controller : Subsystem  TreatAsAtomicUnit=on
  default : Subsystem  TreatAsAtomicUnit=on
  if_below_target_sr : If  IfExpression=u1 == 0
  delta_torque : Outport  VectorParamsAs1DForOutWhenUnconnected=off
  wires:
  Merge/1 -> delta_torque/1
  default/1(no_change) -> Merge/1
  PD Controller/1(delta_torque) -> Merge/2
  dslip/1 -> PD Controller/1(dslip), GreaterThan/1
  enable_tc/1 -> PD Controller/2(enable_tc)
  Kp/1 -> PD Controller/3(Kp)
  Kd/1 -> PD Controller/4(Kd)
  GreaterThan/1 -> if_below_target_sr/1
  Constant/1 -> GreaterThan/2
  if_below_target_sr/1 -> default/Action
  if_below_target_sr/2 -> PD Controller/Action

== system TorqueVect/CarMaker/IPG Vehicle/PowerTrain/PTControl Example/PTControl_ALL_Speedgoat/New TC/TC R3/traction_controller/traction_controller ==
  dslip : Inport
  enable_tc : Inport  Port=2
  Kp : Inport  Port=3
  Kd : Inport  Port=4
  Constant : Constant  Value=0
  GreaterThan : RelationalOperator  Operator=>  OutDataTypeStr=boolean  RndMeth=Simplest  InputSameDT=off
  Merge : Merge
  PD Controller : Subsystem  TreatAsAtomicUnit=on
  default : Subsystem  TreatAsAtomicUnit=on
  if_below_target_sr : If  IfExpression=u1 == 0
  delta_torque : Outport  VectorParamsAs1DForOutWhenUnconnected=off
  wires:
  Merge/1 -> delta_torque/1
  default/1(no_change) -> Merge/1
  PD Controller/1(delta_torque) -> Merge/2
  dslip/1 -> PD Controller/1(dslip), GreaterThan/1
  enable_tc/1 -> PD Controller/2(enable_tc)
  Kp/1 -> PD Controller/3(Kp)
  Kd/1 -> PD Controller/4(Kd)
  GreaterThan/1 -> if_below_target_sr/1
  Constant/1 -> GreaterThan/2
  if_below_target_sr/1 -> default/Action
  if_below_target_sr/2 -> PD Controller/Action

== system TorqueVect/CarMaker/IPG Vehicle/PowerTrain/PTControl Example/PTControl_ALL_Speedgoat/New TC/TC R4/traction_controller/traction_controller ==
  dslip : Inport
  enable_tc : Inport  Port=2
  Kp : Inport  Port=3
  Kd : Inport  Port=4
  Constant : Constant  Value=0
  GreaterThan : RelationalOperator  Operator=>  OutDataTypeStr=boolean  RndMeth=Simplest  InputSameDT=off
  Merge : Merge
  PD Controller : Subsystem  TreatAsAtomicUnit=on
  default : Subsystem  TreatAsAtomicUnit=on
  if_below_target_sr : If  IfExpression=u1 == 0
  delta_torque : Outport  VectorParamsAs1DForOutWhenUnconnected=off
  wires:
  Merge/1 -> delta_torque/1
  default/1(no_change) -> Merge/1
  PD Controller/1(delta_torque) -> Merge/2
  dslip/1 -> PD Controller/1(dslip), GreaterThan/1
  enable_tc/1 -> PD Controller/2(enable_tc)
  Kp/1 -> PD Controller/3(Kp)
  Kd/1 -> PD Controller/4(Kd)
  GreaterThan/1 -> if_below_target_sr/1
  Constant/1 -> GreaterThan/2
  if_below_target_sr/1 -> default/Action
  if_below_target_sr/2 -> PD Controller/Action

== system TorqueVect/CarMaker/IPG Vehicle/PowerTrain/PTControl Example/PTControl_PC_MFE/New TC/TC R1/traction_controller/traction_controller ==
  dslip : Inport
  enable_tc : Inport  Port=2
  Kp : Inport  Port=3
  Kd : Inport  Port=4
  Constant : Constant  Value=0
  GreaterThan : RelationalOperator  Operator=>  OutDataTypeStr=boolean  RndMeth=Simplest  InputSameDT=off
  Merge : Merge
  PD Controller : Subsystem  TreatAsAtomicUnit=on
  default : Subsystem  TreatAsAtomicUnit=on
  if_below_target_sr : If  IfExpression=u1 == 0
  delta_torque : Outport  VectorParamsAs1DForOutWhenUnconnected=off
  wires:
  Merge/1 -> delta_torque/1
  default/1(no_change) -> Merge/1
  PD Controller/1(delta_torque) -> Merge/2
  dslip/1 -> PD Controller/1(dslip), GreaterThan/1
  enable_tc/1 -> PD Controller/2(enable_tc)
  Kp/1 -> PD Controller/3(Kp)
  Kd/1 -> PD Controller/4(Kd)
  GreaterThan/1 -> if_below_target_sr/1
  Constant/1 -> GreaterThan/2
  if_below_target_sr/1 -> default/Action
  if_below_target_sr/2 -> PD Controller/Action

== system TorqueVect/CarMaker/IPG Vehicle/PowerTrain/PTControl Example/PTControl_PC_MFE/New TC/TC R2/traction_controller/traction_controller ==
  dslip : Inport
  enable_tc : Inport  Port=2
  Kp : Inport  Port=3
  Kd : Inport  Port=4
  Constant : Constant  Value=0
  GreaterThan : RelationalOperator  Operator=>  OutDataTypeStr=boolean  RndMeth=Simplest  InputSameDT=off
  Merge : Merge
  PD Controller : Subsystem  TreatAsAtomicUnit=on
  default : Subsystem  TreatAsAtomicUnit=on
  if_below_target_sr : If  IfExpression=u1 == 0
  delta_torque : Outport  VectorParamsAs1DForOutWhenUnconnected=off
  wires:
  Merge/1 -> delta_torque/1
  default/1(no_change) -> Merge/1
  PD Controller/1(delta_torque) -> Merge/2
  dslip/1 -> PD Controller/1(dslip), GreaterThan/1
  enable_tc/1 -> PD Controller/2(enable_tc)
  Kp/1 -> PD Controller/3(Kp)
  Kd/1 -> PD Controller/4(Kd)
  GreaterThan/1 -> if_below_target_sr/1
  Constant/1 -> GreaterThan/2
  if_below_target_sr/1 -> default/Action
  if_below_target_sr/2 -> PD Controller/Action

== system TorqueVect/CarMaker/IPG Vehicle/PowerTrain/PTControl Example/PTControl_PC_MFE/New TC/TC R3/traction_controller/traction_controller ==
  dslip : Inport
  enable_tc : Inport  Port=2
  Kp : Inport  Port=3
  Kd : Inport  Port=4
  Constant : Constant  Value=0
  GreaterThan : RelationalOperator  Operator=>  OutDataTypeStr=boolean  RndMeth=Simplest  InputSameDT=off
  Merge : Merge
  PD Controller : Subsystem  TreatAsAtomicUnit=on
  default : Subsystem  TreatAsAtomicUnit=on
  if_below_target_sr : If  IfExpression=u1 == 0
  delta_torque : Outport  VectorParamsAs1DForOutWhenUnconnected=off
  wires:
  Merge/1 -> delta_torque/1
  default/1(no_change) -> Merge/1
  PD Controller/1(delta_torque) -> Merge/2
  dslip/1 -> PD Controller/1(dslip), GreaterThan/1
  enable_tc/1 -> PD Controller/2(enable_tc)
  Kp/1 -> PD Controller/3(Kp)
  Kd/1 -> PD Controller/4(Kd)
  GreaterThan/1 -> if_below_target_sr/1
  Constant/1 -> GreaterThan/2
  if_below_target_sr/1 -> default/Action
  if_below_target_sr/2 -> PD Controller/Action

== system TorqueVect/CarMaker/IPG Vehicle/PowerTrain/PTControl Example/PTControl_PC_MFE/New TC/TC R4/traction_controller/traction_controller ==
  dslip : Inport
  enable_tc : Inport  Port=2
  Kp : Inport  Port=3
  Kd : Inport  Port=4
  Constant : Constant  Value=0
  GreaterThan : RelationalOperator  Operator=>  OutDataTypeStr=boolean  RndMeth=Simplest  InputSameDT=off
  Merge : Merge
  PD Controller : Subsystem  TreatAsAtomicUnit=on
  default : Subsystem  TreatAsAtomicUnit=on
  if_below_target_sr : If  IfExpression=u1 == 0
  delta_torque : Outport  VectorParamsAs1DForOutWhenUnconnected=off
  wires:
  Merge/1 -> delta_torque/1
  default/1(no_change) -> Merge/1
  PD Controller/1(delta_torque) -> Merge/2
  dslip/1 -> PD Controller/1(dslip), GreaterThan/1
  enable_tc/1 -> PD Controller/2(enable_tc)
  Kp/1 -> PD Controller/3(Kp)
  Kd/1 -> PD Controller/4(Kd)
  GreaterThan/1 -> if_below_target_sr/1
  Constant/1 -> GreaterThan/2
  if_below_target_sr/1 -> default/Action
  if_below_target_sr/2 -> PD Controller/Action

== system TorqueVect/CarMaker/IPG Vehicle/PowerTrain/PTControl Example/PTControl_PC_TC_MFE/New TC/TC R1/traction_controller/traction_controller ==
  dslip : Inport
  enable_tc : Inport  Port=2
  Kp : Inport  Port=3
  Kd : Inport  Port=4
  Constant : Constant  Value=0
  GreaterThan : RelationalOperator  Operator=>  OutDataTypeStr=boolean  RndMeth=Simplest  InputSameDT=off
  Merge : Merge
  PD Controller : Subsystem  TreatAsAtomicUnit=on
  default : Subsystem  TreatAsAtomicUnit=on
  if_below_target_sr : If  IfExpression=u1 == 0
  delta_torque : Outport  VectorParamsAs1DForOutWhenUnconnected=off
  wires:
  Merge/1 -> delta_torque/1
  default/1(no_change) -> Merge/1
  PD Controller/1(delta_torque) -> Merge/2
  dslip/1 -> PD Controller/1(dslip), GreaterThan/1
  enable_tc/1 -> PD Controller/2(enable_tc)
  Kp/1 -> PD Controller/3(Kp)
  Kd/1 -> PD Controller/4(Kd)
  GreaterThan/1 -> if_below_target_sr/1
  Constant/1 -> GreaterThan/2
  if_below_target_sr/1 -> default/Action
  if_below_target_sr/2 -> PD Controller/Action

== system TorqueVect/CarMaker/IPG Vehicle/PowerTrain/PTControl Example/PTControl_PC_TC_MFE/New TC/TC R2/traction_controller/traction_controller ==
  dslip : Inport
  enable_tc : Inport  Port=2
  Kp : Inport  Port=3
  Kd : Inport  Port=4
  Constant : Constant  Value=0
  GreaterThan : RelationalOperator  Operator=>  OutDataTypeStr=boolean  RndMeth=Simplest  InputSameDT=off
  Merge : Merge
  PD Controller : Subsystem  TreatAsAtomicUnit=on
  default : Subsystem  TreatAsAtomicUnit=on
  if_below_target_sr : If  IfExpression=u1 == 0
  delta_torque : Outport  VectorParamsAs1DForOutWhenUnconnected=off
  wires:
  Merge/1 -> delta_torque/1
  default/1(no_change) -> Merge/1
  PD Controller/1(delta_torque) -> Merge/2
  dslip/1 -> PD Controller/1(dslip), GreaterThan/1
  enable_tc/1 -> PD Controller/2(enable_tc)
  Kp/1 -> PD Controller/3(Kp)
  Kd/1 -> PD Controller/4(Kd)
  GreaterThan/1 -> if_below_target_sr/1
  Constant/1 -> GreaterThan/2
  if_below_target_sr/1 -> default/Action
  if_below_target_sr/2 -> PD Controller/Action

== system TorqueVect/CarMaker/IPG Vehicle/PowerTrain/PTControl Example/PTControl_PC_TC_MFE/New TC/TC R3/traction_controller/traction_controller ==
  dslip : Inport
  enable_tc : Inport  Port=2
  Kp : Inport  Port=3
  Kd : Inport  Port=4
  Constant : Constant  Value=0
  GreaterThan : RelationalOperator  Operator=>  OutDataTypeStr=boolean  RndMeth=Simplest  InputSameDT=off
  Merge : Merge
  PD Controller : Subsystem  TreatAsAtomicUnit=on
  default : Subsystem  TreatAsAtomicUnit=on
  if_below_target_sr : If  IfExpression=u1 == 0
  delta_torque : Outport  VectorParamsAs1DForOutWhenUnconnected=off
  wires:
  Merge/1 -> delta_torque/1
  default/1(no_change) -> Merge/1
  PD Controller/1(delta_torque) -> Merge/2
  dslip/1 -> PD Controller/1(dslip), GreaterThan/1
  enable_tc/1 -> PD Controller/2(enable_tc)
  Kp/1 -> PD Controller/3(Kp)
  Kd/1 -> PD Controller/4(Kd)
  GreaterThan/1 -> if_below_target_sr/1
  Constant/1 -> GreaterThan/2
  if_below_target_sr/1 -> default/Action
  if_below_target_sr/2 -> PD Controller/Action

== system TorqueVect/CarMaker/IPG Vehicle/PowerTrain/PTControl Example/PTControl_PC_TC_MFE/New TC/TC R4/traction_controller/traction_controller ==
  dslip : Inport
  enable_tc : Inport  Port=2
  Kp : Inport  Port=3
  Kd : Inport  Port=4
  Constant : Constant  Value=0
  GreaterThan : RelationalOperator  Operator=>  OutDataTypeStr=boolean  RndMeth=Simplest  InputSameDT=off
  Merge : Merge
  PD Controller : Subsystem  TreatAsAtomicUnit=on
  default : Subsystem  TreatAsAtomicUnit=on
  if_below_target_sr : If  IfExpression=u1 == 0
  delta_torque : Outport  VectorParamsAs1DForOutWhenUnconnected=off
  wires:
  Merge/1 -> delta_torque/1
  default/1(no_change) -> Merge/1
  PD Controller/1(delta_torque) -> Merge/2
  dslip/1 -> PD Controller/1(dslip), GreaterThan/1
  enable_tc/1 -> PD Controller/2(enable_tc)
  Kp/1 -> PD Controller/3(Kp)
  Kd/1 -> PD Controller/4(Kd)
  GreaterThan/1 -> if_below_target_sr/1
  Constant/1 -> GreaterThan/2
  if_below_target_sr/1 -> default/Action
  if_below_target_sr/2 -> PD Controller/Action
